simulink model "cpm_jap_r2019a"  (R2019a)
settings: Solver=ode4  StartTime=0.0  StopTime=inf  FixedStep=StepSize  RelTol=1e-3  EnableMultiTasking=on
PostLoadFcn:
  | %% PARAMETER INITIALIZATION
  | modelname = gcs;
  | p = Simulink.Mask.get([modelname, '/CP Model']);
  | 
  | %% HEART
  | % Basal heart period, T0 (s):
  | p.Parameters(1,1).Value = '0.58';
  | %% Right atrium
  | % RA Compliance, Cra (ml/mmHg):
  | p.Parameters(1,2).Value = '31.25';
  | % RA Resistance, Rra (mmHg s/ml):
  | p.Parameters(1,3).Value = '0.0025';
  | % RA Unstressed volume, Vu_ra (ml):
  | p.Parameters(1,4).Value = '22';
  | %% Left atrium
  | % LA Compliance, Cla (ml/mmHg):
  | p.Parameters(1,5).Value = '19.23';
  | % LA Resistance, Rla (mmHg s/ml):
  | p.Parameters(1,6).Value = '0.0025';
  | % LA Unstressed volume, Vu_la (ml):
  | p.Parameters(1,7).Value = '22';
  | %% Right ventricle
  | % RV Resistance coefficient, kR_rv (s/ml):
  | p.Parameters(1,8).Value = '0.0014';
  | % RV free wall End-systolic maximal elastance, Emax_rvf0 (mmHg/ml):
  | p.Parameters(1,9).Value = '1.412';
  | % RV free wall End-systolic unstressed volume, Vu_rvf (ml):
  | p.Parameters(1,10).Value = '35.904';
  | % RV free wall End-diastolic pressure intercept, P0_rvf (mmHg):
  | p.Parameters(1,11).Value = '1.5';
  | % RV free wall End-diastolic elastance coefficient, kE_rvf (1/ml):
  | p.Parameters(1,12).Value = '0.011';
  | % RV free wall Contraction delay (s):
  | p.Parameters(1,13).Value = '0';
  | %% Left ventricle
  | % LV Resistance coefficient, kR_lv (s/ml):
  | p.Parameters(1,14).Value = '0.00037';
  | % LV free wall End-systolic maximal elastance, Emax_lvf0 (mmHg/ml):
  | p.Parameters(1,15).Value = '2.392';
  | % LV free wall End-systolic unstressed volume, Vu_lvf (ml):
  | p.Parameters(1,16).Value = '14.7576';
  | % LV free wall End-diastolic pressure intercept, P0_lvf (mmHg):
  | p.Parameters(1,17).Value = '1.5';
  | % LV free wall End-diastolic elastance coefficient, kE_lvf (1/ml):
  | p.Parameters(1,18).Value = '0.014';
  | % LV Contraction delay (s):
  | p.Parameters(1,19).Value = '0';
  | %% Septum
  | % Septal End-systolic maximal elastance, Emax_spt0 (mmHg/ml):
  | p.Parameters(1,20).Value = '32.4';
  | % Septal End-systolic unstressed volume, Vu_spt (ml):
  | p.Parameters(1,21).Value = '0';
  | % Septal End-diastolic pressure intercept, P0_spt (mmHg):
  | p.Parameters(1,22).Value = '1.11';
  | % Septal End-diastolic elastance coefficient, kE_spt (1/ml):
  | p.Parameters(1,23).Value = '0.175';
  | %% Pericardium
  | % Pericardial Unstressed volume, Vu_pcd (ml):
  | p.Parameters(1,24).Value = '200';
  | % Pericardial Pressure intercept, P0_pcd (mmHg):
  | ... (+188 lines)
InitFcn:
  | logFreq = 100; % logging frequency
  | StepSize = 5e-4; % simulation step size
  | 
  | %% PARAMETER INITIALIZATION
  | modelname = gcs;
  | p = Simulink.Mask.get([modelname, '/CP Model']);
  | 
  | %% HEART
  | % Basal heart period, T0 (s):
  | p.Parameters(1,1).Value = '0.58';
  | %% Right atrium
  | % RA Compliance, Cra (ml/mmHg):
  | p.Parameters(1,2).Value = '31.25';
  | % RA Resistance, Rra (mmHg s/ml):
  | p.Parameters(1,3).Value = '0.0025';
  | % RA Unstressed volume, Vu_ra (ml):
  | p.Parameters(1,4).Value = '22';
  | %% Left atrium
  | % LA Compliance, Cla (ml/mmHg):
  | p.Parameters(1,5).Value = '19.23';
  | % LA Resistance, Rla (mmHg s/ml):
  | p.Parameters(1,6).Value = '0.0025';
  | % LA Unstressed volume, Vu_la (ml):
  | p.Parameters(1,7).Value = '22';
  | %% Right ventricle
  | % RV Resistance coefficient, kR_rv (s/ml):
  | p.Parameters(1,8).Value = '0.0014';
  | % RV free wall End-systolic maximal elastance, Emax_rvf0 (mmHg/ml):
  | p.Parameters(1,9).Value = '1.412';
  | % RV free wall End-systolic unstressed volume, Vu_rvf (ml):
  | p.Parameters(1,10).Value = '35.904';
  | % RV free wall End-diastolic pressure intercept, P0_rvf (mmHg):
  | p.Parameters(1,11).Value = '1.5';
  | % RV free wall End-diastolic elastance coefficient, kE_rvf (1/ml):
  | p.Parameters(1,12).Value = '0.011';
  | % RV free wall Contraction delay (s):
  | p.Parameters(1,13).Value = '0';
  | %% Left ventricle
  | % LV Resistance coefficient, kR_lv (s/ml):
  | p.Parameters(1,14).Value = '0.00037';
  | % LV free wall End-systolic maximal elastance, Emax_lvf0 (mmHg/ml):
  | p.Parameters(1,15).Value = '2.392';
  | % LV free wall End-systolic unstressed volume, Vu_lvf (ml):
  | p.Parameters(1,16).Value = '14.7576';
  | % LV free wall End-diastolic pressure intercept, P0_lvf (mmHg):
  | p.Parameters(1,17).Value = '1.5';
  | % LV free wall End-diastolic elastance coefficient, kE_lvf (1/ml):
  | p.Parameters(1,18).Value = '0.014';
  | % LV Contraction delay (s):
  | p.Parameters(1,19).Value = '0';
  | %% Septum
  | % Septal End-systolic maximal elastance, Emax_spt0 (mmHg/ml):
  | p.Parameters(1,20).Value = '32.4';
  | % Septal End-systolic unstressed volume, Vu_spt (ml):
  | p.Parameters(1,21).Value = '0';
  | % Septal End-diastolic pressure intercept, P0_spt (mmHg):
  | p.Parameters(1,22).Value = '1.11';
  | % Septal End-diastolic elastance coefficient, kE_spt (1/ml):
  | p.Parameters(1,23).Value = '0.175';
  | %% Pericardium
  | ... (+191 lines)
StopFcn:
  | cpmResults = cpm_jap{1}.Values;
(part 2 of 2)

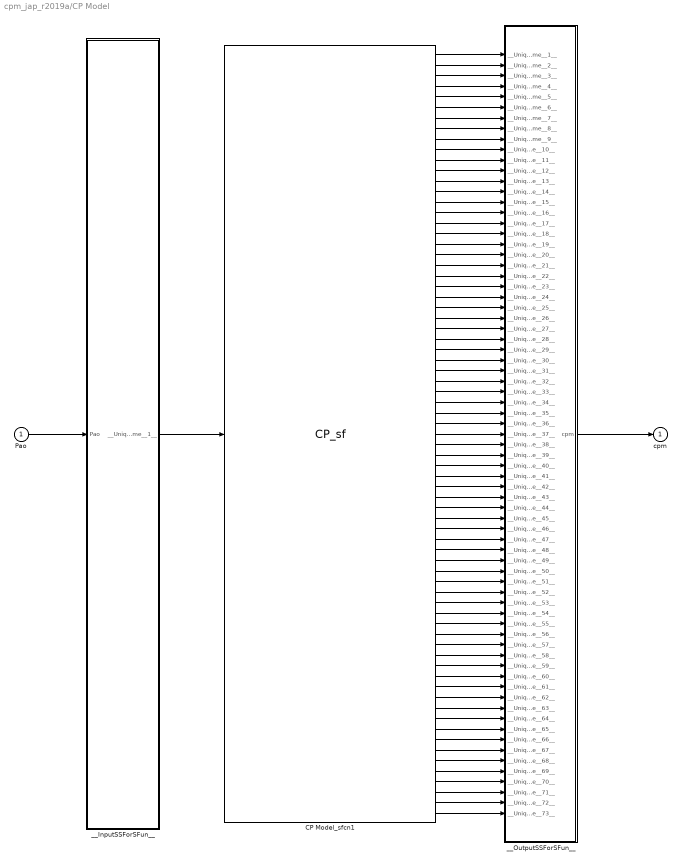
== system cpm_jap_r2019a/CP Model ==
  Pao : Inport  Unit=cmH2O
  CP Model_sfcn1 : S-Function  FunctionName=CP_sf  Parameters=sfcnParam1, sfcnParam2, sfcnParam3, sfcnParam4, sfcnParam5, sfcnParam6, sfcnParam7, sfcnParam8, sfcnParam9, sfcnParam10, sfcnParam11, sfcnParam12, sfcnParam13, sfcnParam14, sfcnParam15, sfcnParam16, sfcnParam17, sfcnParam18, sfcnParam19, sfcnParam20, sfcnParam21, sfcnParam22, sfcnParam23, sfcnParam24, sfcnParam25, sfcnParam26, sfcnParam27, sfcnParam28, sfcnParam29, sfcnParam30, sfcnParam31, sfcnParam32, sfcnParam33, sfcnParam34, sfcnParam35, sfcnParam36, sfcnParam37, sfcnParam38, sfcnParam39, sfcnParam40, sfcnParam41, sfcnParam42, sfcnParam43, sfcnParam44, sfcnParam45, sfcnParam46, sfcnParam47, sfcnParam48, sfcnParam49, sfcnParam50, sfcnParam51, sfcnParam52, sfcnParam53, sfcnParam54, sfcnParam55, sfcnParam56, sfcnParam57, sfcnParam58, sfcnParam59, sfcnParam60, sfcnParam61, sfcnParam62, sfcnParam63, sfcnParam64, sfcnParam65, sfcnParam66, sfcnParam67, sfcnParam68, sfcnParam69, sfcnParam70, sfcnParam71, sfcnParam72, sfcnParam73, sfcnParam74, sfcnParam75, sfcnParam76, sfcnParam77, sfcnParam78, sfcnParam79, sfcnParam80, sfcnParam81, sfcnParam82, sfcnParam83, sfcnParam84, sfcnParam85, sfcnParam86, sfcnParam87, sfcnParam88, sfcnParam89, sfcnParam90, sfcnParam91, sfcnParam92, sfcnParam93, sfcnParam94, sfcnParam95, sfcnParam96, sfcnParam97, sfcnParam98, sfcnParam99, sfcnParam100, sfcnParam101, sfcnParam102, sfcnParam103, sfcnParam104, sfcnParam105, sfcnParam106, sfcnParam107, sfcnParam108, sfcnParam109, sfcnParam110, sfcnParam111  SFunctionModules=""  SFunctionDeploymentMode=off  EnableBusSupport=off  SFcnStateName=DWORK0  mask{rtw_sf_name=CP_sf, showVar=off, sfcnParam1=sfcnParam1, sfcnParam2=sfcnParam2, sfcnParam3=sfcnParam3, sfcnParam4=sfcnParam4, sfcnParam5=sfcnParam5, sfcnParam6=sfcnParam6, sfcnParam7=sfcnParam7, sfcnParam8=sfcnParam8, sfcnParam9=sfcnParam9, sfcnParam10=sfcnParam10, sfcnParam11=sfcnParam11, sfcnParam12=sfcnParam12, sfcnParam13=sfcnParam13, sfcnParam14=sfcnParam14, sfcnParam15=sfcnParam15, sfcnParam16=sfcnParam16, sfcnParam17=sfcnParam17, sfcnParam18=sfcnParam18, sfcnParam19=sfcnParam19, sfcnParam20=sfcnParam20, sfcnParam21=sfcnParam21, sfcnParam22=sfcnParam22, sfcnParam23=sfcnParam23, sfcnParam24=2.25, sfcnParam25=sfcnParam25, sfcnParam26=sfcnParam26, sfcnParam27=sfcnParam27, sfcnParam28=sfcnParam28, sfcnParam29=sfcnParam29, sfcnParam30=sfcnParam30, sfcnParam31=sfcnParam31, sfcnParam32=sfcnParam32, sfcnParam33=sfcnParam33, sfcnParam34=sfcnParam34, sfcnParam35=sfcnParam35, sfcnParam36=sfcnParam36, sfcnParam37=sfcnParam37, sfcnParam38=sfcnParam38, sfcnParam39=sfcnParam39, sfcnParam40=sfcnParam40, sfcnParam41=sfcnParam41, sfcnParam42=sfcnParam42, sfcnParam43=sfcnParam43, sfcnParam44=sfcnParam44, sfcnParam45=sfcnParam45, sfcnParam46=sfcnParam46, sfcnParam47=sfcnParam47, sfcnParam48=sfcnParam48, sfcnParam49=sfcnParam49, sfcnParam50=sfcnParam50, sfcnParam51=sfcnParam51, sfcnParam52=sfcnParam52, sfcnParam53=sfcnParam53, sfcnParam54=sfcnParam54, sfcnParam55=sfcnParam55, sfcnParam56=sfcnParam56, sfcnParam57=sfcnParam57, sfcnParam58=sfcnParam58, sfcnParam59=sfcnParam59, sfcnParam60=sfcnParam60, sfcnParam61=sfcnParam61, sfcnParam62=sfcnParam62, sfcnParam63=sfcnParam63, sfcnParam64=sfcnParam64, sfcnParam65=sfcnParam65, sfcnParam66=sfcnParam66, sfcnParam67=sfcnParam67, sfcnParam68=sfcnParam68, sfcnParam69=sfcnParam69, sfcnParam70=sfcnParam70, sfcnParam71=sfcnParam71, sfcnParam72=0, sfcnParam73=sfcnParam73, sfcnParam74=sfcnParam74, sfcnParam75=sfcnParam75, sfcnParam76=sfcnParam76, sfcnParam77=sfcnParam77, sfcnParam78=sfcnParam78, sfcnParam79=sfcnParam79, sfcnParam80=sfcnParam80, sfcnParam81=sfcnParam81, sfcnParam82=sfcnParam82, sfcnParam83=sfcnParam83, sfcnParam84=sfcnParam84, sfcnParam85=sfcnParam85, sfcnParam86=sfcnParam86, sfcnParam87=sfcnParam87, sfcnParam88=sfcnParam88, sfcnParam89=sfcnParam89, sfcnParam90=sfcnParam90, sfcnParam91=sfcnParam91, sfcnParam92=sfcnParam92, sfcnParam93=sfcnParam93, sfcnParam94=sfcnParam94, sfcnParam95=sfcnParam95, sfcnParam96=0, sfcnParam97=sfcnParam97, sfcnParam98=sfcnParam98, sfcnParam99=sfcnParam99, sfcnParam100=sfcnParam100, sfcnParam101=sfcnParam101, sfcnParam102=sfcnParam102, sfcnParam103=sfcnParam103, sfcnParam104=sfcnParam104, sfcnParam105=sfcnParam105, sfcnParam106=sfcnParam106, sfcnParam107=sfcnParam107, sfcnParam108=sfcnParam108, sfcnParam109=sfcnParam109, sfcnParam110=sfcnParam110, sfcnParam111=sfcnParam111}
      mask prompts: rtw_sf_name "Simulink:masks:GenSFuncName_MP"; showVar "Simulink:masks:GenSFuncShowModuleList_MP"; sfcnParam1 "BreathAmp:"; sfcnParam2 "BreathFreq:"; sfcnParam3 "CL:"; sfcnParam4 "C_cw:"; sfcnParam5 "C_vc:"; sfcnParam6 "Cep:"; sfcnParam7 "Cev:"; sfcnParam8 "Cla:"; sfcnParam9 "ConsCO2Exspl:"; sfcnParam10 "ConsCO2Spl:"; sfcnParam11 "ConsO2Exspl:"; sfcnParam12 "ConsO2Spl:"; sfcnParam13 "Cpa:"; sfcnParam14 "Cpp_tot:"; sfcnParam15 "Cpv:"; sfcnParam16 "Cra:"; sfcnParam17 "Csa:"; sfcnParam18 "Csp:"; sfcnParam19 "Csv:"; sfcnParam20 "Ees_spt0:"; sfcnParam21 "Emax_lvf0:"; sfcnParam22 "Emax_rvf0:"; sfcnParam23 "ExsplVolume:"; sfcnParam24 "FRCnom:"; sfcnParam25 "FiCO2:"; sfcnParam26 "FiO2:"; sfcnParam27 "Gc_A_up:"; sfcnParam28 "Gc_f_up:"; sfcnParam29 "Gp_A_up:"; sfcnParam30 "Gp_f_up:"; sfcnParam31 "Gsr:"; sfcnParam32 "IEratio:"; sfcnParam33 "Lpa:"; sfcnParam34 "Lsa:"; sfcnParam35 "P0_lvf:"; sfcnParam36 "P0_pcd:"; sfcnParam37 "P0_rvf:"; sfcnParam38 "P0_spt:"; sfcnParam39 "PO2sh:"; sfcnParam40 "PO2sp:"; sfcnParam41 "PO2sv:"; sfcnParam42 "PaCO2n:"; sfcnParam43 "Pn:"; sfcnParam44 "RL:"; sfcnParam45 "R_vc_0:"; sfcnParam46 "Rep_0:"; sfcnParam47 "Ret:"; sfcnParam48 "Rev:"; sfcnParam49 "Rla:"; sfcnParam50 "Rpa:"; sfcnParam51 "Rpp_tot:"; sfcnParam52 "Rpv:"; sfcnParam53 "Rra:"; sfcnParam54 "Rsa:"; sfcnParam55 "Rsp_0:"; sfcnParam56 "Rsv:"; sfcnParam57 "SplVolume:"; sfcnParam58 "T0:"; sfcnParam59 "V0_pcd:"; sfcnParam60 "V0_spt:"; sfcnParam61 "V_pcd:"; sfcnParam62 "Vdead:"; sfcnParam63 "Vt:"; sfcnParam64 "Vu_L:"; sfcnParam65 "Vu_cw:"; sfcnParam66 "Vu_ep:"; sfcnParam67 "Vu_ev0:"; sfcnParam68 "Vu_la:"; sfcnParam69 "Vu_lvf:"; sfcnParam70 "Vu_pa:"; sfcnParam71 "Vu_pp:"; sfcnParam72 "Vu_ps:"; sfcnParam73 "Vu_pv:"; sfcnParam74 "Vu_ra:"; sfcnParam75 "Vu_rvf:"; sfcnParam76 "Vu_sa:"; sfcnParam77 "Vu_sp:"; sfcnParam78 "Vu_sv0:"; sfcnParam79 "Vu_vc:"; sfcnParam80 "Wbsh:"; sfcnParam81 "Wbsp:"; sfcnParam82 "Wbsv:"; sfcnParam83 "Wpcsh:"; sfcnParam84 "Wpcsp:"; sfcnParam85 "Wpcsv:"; sfcnParam86 "Wpcv:"; sfcnParam87 "Wsrsh:"; sfcnParam88 "Wsrsp:"; sfcnParam89 "Wsrsv:"; sfcnParam90 "Wsrv:"; sfcnParam91 "fapcn:"; sfcnParam92 "gccsh:"; sfcnParam93 "gccsp:"; sfcnParam94 "gccsv:"; sfcnParam95 "infusionDur:"; sfcnParam96 "kBloodLoss:"; sfcnParam97 "kE_lvf:"; sfcnParam98 "kE_rvf:"; sfcnParam99 "kRL_out:"; sfcnParam100 "kR_lv:"; sfcnParam101 "kR_rv:"; sfcnParam102 "kab:"; sfcnParam103 "kev:"; sfcnParam104 "lambda_pcd:"; sfcnParam105 "lambda_spt:"; sfcnParam106 "lvContractionDelay:"; sfcnParam107 "passivePatient:"; sfcnParam108 "pumpFlag:"; sfcnParam109 "rvContractionDelay:"; sfcnParam110 "sh:"; sfcnParam111 "volumeInfused:"
      mask help: Simulink:masks:GenSFuncDesc_MD
      mask init:
      | displist = '';
      | if ~strcmp(get_param(gcb, 'FunctionName'), rtw_sf_name);
      |   set_param(gcb, 'FunctionName', rtw_sf_name);
      | end
      | % Check if we are generating code
      | rtw_mode = false;
      | if strcmpi(get_param(bdroot(gcb),'SimulationStatus'),'Initializing')
      | 	rtw_mode = strcmpi(get_param(bdroot(gcb),'BuildingRTWCode'),'on') && ...
      | 		~strcmpi(get_param(bdroot(gcb),'TargetStyle'),'SimulationTarget');
      | end
      | if showVar || rtw_mode
      | 	if exist('rtwsfunc') == 2 | exist('rtwsfunc') == 6
      | 		tmplist = rtwsfunc(rtw_sf_name,gcb);
      | 		tmplist = DAStudio.message('Simulink:masks:GenSFuncListOfModules_IC', tmplist);
      | 	elseif showVar
      | 		tmplist1 = DAStudio.message('Simulink:masks:GenSFuncListOfModules_IC', '');
      |         tmplist2 = DAStudio.message('Simulink:masks:GenSFuncNotLicensed_IC');
      |         tmplist = [tmplist1 tmplist2];
      |  	end
      | end
      | if showVar
      |   displist = tmplist;
      | end
      settings: SFcnIsStateOwnerBlock=on
      settings: CopyFcn=|
      | if ~strcmp(get_param(gcb,'Linkstatus'),'none') && ...
      | ~strcmp(get_param(gcb,'Linkstatus'),'implicit')
      |   set_param(gcb,'LinkStatus','none');
      | end
      mask Help: eval('feval(''rtwprivate'',''rtwhelpview'',''rtw_sfcn_block'')');
      mask Display:
      | port_label('input',1,'Pao');
      | port_label('output',1,'Air flow');
      | port_label('output',2,'Pmus');
      | port_label('output',3,'Pao');
      | port_label('output',4,'PA');
      | port_label('output',5,'Ppl');
      | port_label('output',6,'V_T');
      | port_label('output',7,'V_L');
      | port_label('output',8,'Ve');
      | port_label('output',9,'RR');
      | port_label('output',10,'WOB');
      | port_label('output',11,'POB');
      | port_label('output',12,'PaO2');
      | port_label('output',13,'PaCO2');
      | port_label('output',14,'PAO2');
      | port_label('output',15,'PACO2');
      | port_label('output',16,'SaO2');
      | port_label('output',17,'ETCO2');
      | port_label('output',18,'fab');
      | port_label('output',19,'fapc');
      | port_label('output',20,'fasr');
      | port_label('output',21,'fsh');
      | port_label('output',22,'fsp');
      | port_label('output',23,'fsv');
      | port_label('output',24,'fev');
      | port_label('output',25,'Psa');
      | port_label('output',26,'Psa_sys');
      | port_label('output',27,'Psa_dias');
      | port_label('output',28,'Psa_mean');
      | port_label('output',29,'PP');
      | port_label('output',30,'DPP');
      | port_label('output',31,'Ppa');
      | port_label('output',32,'Ppa_sys');
      | port_label('output',33,'Ppa_dias');
      | port_label('output',34,'Ppa_mean');
      | port_label('output',35,'Pla');
      | port_label('output',36,'Pra');
      | port_label('output',37,'Plv');
      | port_label('output',38,'Prv');
      | port_label('output',39,'CO');
      | port_label('output',40,'CO_mean');
      | port_label('output',41,'HR');
      | port_label('output',42,'HR_mean');
      | port_label('output',43,'SV');
      | port_label('output',44,'SV_mean');
      | port_label('output',45,'SVI');
      | port_label('output',46,'SVI_mean');
      | port_label('output',47,'CI');
      | port_label('output',48,'CI_mean');
      | port_label('output',49,'phi');
      | port_label('output',50,'Vlv');
      | port_label('output',51,'Vlvf');
      | port_label('output',52,'Vrv');
      | port_label('output',53,'Vrvf');
      | port_label('output',54,'LVEF');
      | port_label('output',55,'LVESV');
      | port_label('output',56,'LVEDV');
      | port_label('output',57,'RVEF');
      | port_label('output',58,'RVESV');
      | port_label('output',59,'RVEDV');
      | port_label('output',60,'Qlvo');
      | port_label('output',61,'Qrvo');
      | port_label('output',62,'Pperi');
      | port_label('output',63,'Vspt');
      | port_label('output',64,'Vblood_thorax');
      | port_label('output',65,'Vblood_t');
      | port_label('output',66,'Emax_rvf');
      | port_label('output',67,'Emax_lvf');
      | port_label('output',68,'Emax_spt');
      | port_label('output',69,'Rsp');
      | port_label('output',70,'Rep');
      | port_label('output',71,'Vu_sv');
      | port_label('output',72,'Vu_ev');
      | port_label('output',73,'T');
  __InputSSForSFun__ : Subsystem
  __OutputSSForSFun__ : Subsystem
  cpm : Outport
  wires:
  Pao/1 -> __InputSSForSFun__/1(Pao)
  __InputSSForSFun__/1(__UniqueOutportName__1__) -> CP Model_sfcn1/1
  CP Model_sfcn1/1 -> __OutputSSForSFun__/1(__UniqueInportName__1__)
  CP Model_sfcn1/2 -> __OutputSSForSFun__/2(__UniqueInportName__2__)
  CP Model_sfcn1/3 -> __OutputSSForSFun__/3(__UniqueInportName__3__)
  CP Model_sfcn1/4 -> __OutputSSForSFun__/4(__UniqueInportName__4__)
  CP Model_sfcn1/5 -> __OutputSSForSFun__/5(__UniqueInportName__5__)
  CP Model_sfcn1/6 -> __OutputSSForSFun__/6(__UniqueInportName__6__)
  CP Model_sfcn1/7 -> __OutputSSForSFun__/7(__UniqueInportName__7__)
  CP Model_sfcn1/8 -> __OutputSSForSFun__/8(__UniqueInportName__8__)
  CP Model_sfcn1/9 -> __OutputSSForSFun__/9(__UniqueInportName__9__)
  CP Model_sfcn1/10 -> __OutputSSForSFun__/10(__UniqueInportName__10__)
  CP Model_sfcn1/11 -> __OutputSSForSFun__/11(__UniqueInportName__11__)
  CP Model_sfcn1/12 -> __OutputSSForSFun__/12(__UniqueInportName__12__)
  CP Model_sfcn1/13 -> __OutputSSForSFun__/13(__UniqueInportName__13__)
  CP Model_sfcn1/14 -> __OutputSSForSFun__/14(__UniqueInportName__14__)
  CP Model_sfcn1/15 -> __OutputSSForSFun__/15(__UniqueInportName__15__)
  CP Model_sfcn1/16 -> __OutputSSForSFun__/16(__UniqueInportName__16__)
  CP Model_sfcn1/17 -> __OutputSSForSFun__/17(__UniqueInportName__17__)
  CP Model_sfcn1/18 -> __OutputSSForSFun__/18(__UniqueInportName__18__)
  CP Model_sfcn1/19 -> __OutputSSForSFun__/19(__UniqueInportName__19__)
  CP Model_sfcn1/20 -> __OutputSSForSFun__/20(__UniqueInportName__20__)
  CP Model_sfcn1/21 -> __OutputSSForSFun__/21(__UniqueInportName__21__)
  CP Model_sfcn1/22 -> __OutputSSForSFun__/22(__UniqueInportName__22__)
  CP Model_sfcn1/23 -> __OutputSSForSFun__/23(__UniqueInportName__23__)
  CP Model_sfcn1/24 -> __OutputSSForSFun__/24(__UniqueInportName__24__)
  CP Model_sfcn1/25 -> __OutputSSForSFun__/25(__UniqueInportName__25__)
  CP Model_sfcn1/26 -> __OutputSSForSFun__/26(__UniqueInportName__26__)
  CP Model_sfcn1/27 -> __OutputSSForSFun__/27(__UniqueInportName__27__)
  CP Model_sfcn1/28 -> __OutputSSForSFun__/28(__UniqueInportName__28__)
  CP Model_sfcn1/29 -> __OutputSSForSFun__/29(__UniqueInportName__29__)
  CP Model_sfcn1/30 -> __OutputSSForSFun__/30(__UniqueInportName__30__)
  CP Model_sfcn1/31 -> __OutputSSForSFun__/31(__UniqueInportName__31__)
  CP Model_sfcn1/32 -> __OutputSSForSFun__/32(__UniqueInportName__32__)
  CP Model_sfcn1/33 -> __OutputSSForSFun__/33(__UniqueInportName__33__)
  CP Model_sfcn1/34 -> __OutputSSForSFun__/34(__UniqueInportName__34__)
  CP Model_sfcn1/35 -> __OutputSSForSFun__/35(__UniqueInportName__35__)
  CP Model_sfcn1/36 -> __OutputSSForSFun__/36(__UniqueInportName__36__)
  CP Model_sfcn1/37 -> __OutputSSForSFun__/37(__UniqueInportName__37__)
  CP Model_sfcn1/38 -> __OutputSSForSFun__/38(__UniqueInportName__38__)
  CP Model_sfcn1/39 -> __OutputSSForSFun__/39(__UniqueInportName__39__)
  CP Model_sfcn1/40 -> __OutputSSForSFun__/40(__UniqueInportName__40__)
  CP Model_sfcn1/41 -> __OutputSSForSFun__/41(__UniqueInportName__41__)
  CP Model_sfcn1/42 -> __OutputSSForSFun__/42(__UniqueInportName__42__)
  CP Model_sfcn1/43 -> __OutputSSForSFun__/43(__UniqueInportName__43__)
  CP Model_sfcn1/44 -> __OutputSSForSFun__/44(__UniqueInportName__44__)
  CP Model_sfcn1/45 -> __OutputSSForSFun__/45(__UniqueInportName__45__)
  CP Model_sfcn1/46 -> __OutputSSForSFun__/46(__UniqueInportName__46__)
  CP Model_sfcn1/47 -> __OutputSSForSFun__/47(__UniqueInportName__47__)
  CP Model_sfcn1/48 -> __OutputSSForSFun__/48(__UniqueInportName__48__)
  CP Model_sfcn1/49 -> __OutputSSForSFun__/49(__UniqueInportName__49__)
  CP Model_sfcn1/50 -> __OutputSSForSFun__/50(__UniqueInportName__50__)
  CP Model_sfcn1/51 -> __OutputSSForSFun__/51(__UniqueInportName__51__)
  CP Model_sfcn1/52 -> __OutputSSForSFun__/52(__UniqueInportName__52__)
  CP Model_sfcn1/53 -> __OutputSSForSFun__/53(__UniqueInportName__53__)
  CP Model_sfcn1/54 -> __OutputSSForSFun__/54(__UniqueInportName__54__)
  CP Model_sfcn1/55 -> __OutputSSForSFun__/55(__UniqueInportName__55__)
  CP Model_sfcn1/56 -> __OutputSSForSFun__/56(__UniqueInportName__56__)
  CP Model_sfcn1/57 -> __OutputSSForSFun__/57(__UniqueInportName__57__)
  CP Model_sfcn1/58 -> __OutputSSForSFun__/58(__UniqueInportName__58__)
  CP Model_sfcn1/59 -> __OutputSSForSFun__/59(__UniqueInportName__59__)
  CP Model_sfcn1/60 -> __OutputSSForSFun__/60(__UniqueInportName__60__)
  CP Model_sfcn1/61 -> __OutputSSForSFun__/61(__UniqueInportName__61__)
  CP Model_sfcn1/62 -> __OutputSSForSFun__/62(__UniqueInportName__62__)
  CP Model_sfcn1/63 -> __OutputSSForSFun__/63(__UniqueInportName__63__)
  CP Model_sfcn1/64 -> __OutputSSForSFun__/64(__UniqueInportName__64__)
  CP Model_sfcn1/65 -> __OutputSSForSFun__/65(__UniqueInportName__65__)
  CP Model_sfcn1/66 -> __OutputSSForSFun__/66(__UniqueInportName__66__)
  CP Model_sfcn1/67 -> __OutputSSForSFun__/67(__UniqueInportName__67__)
  CP Model_sfcn1/68 -> __OutputSSForSFun__/68(__UniqueInportName__68__)
  CP Model_sfcn1/69 -> __OutputSSForSFun__/69(__UniqueInportName__69__)
  CP Model_sfcn1/70 -> __OutputSSForSFun__/70(__UniqueInportName__70__)
  CP Model_sfcn1/71 -> __OutputSSForSFun__/71(__UniqueInportName__71__)
  CP Model_sfcn1/72 -> __OutputSSForSFun__/72(__UniqueInportName__72__)
  CP Model_sfcn1/73 -> __OutputSSForSFun__/73(__UniqueInportName__73__)
  __OutputSSForSFun__/1(cpm) -> cpm/1

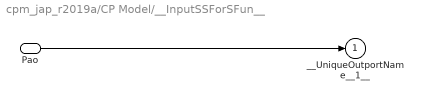
== system cpm_jap_r2019a/CP Model/__InputSSForSFun__ ==
  Pao : Inport  Unit=cmH2O
  __UniqueOutportName__1__ : Outport
  wires:
  Pao/1 -> __UniqueOutportName__1__/1

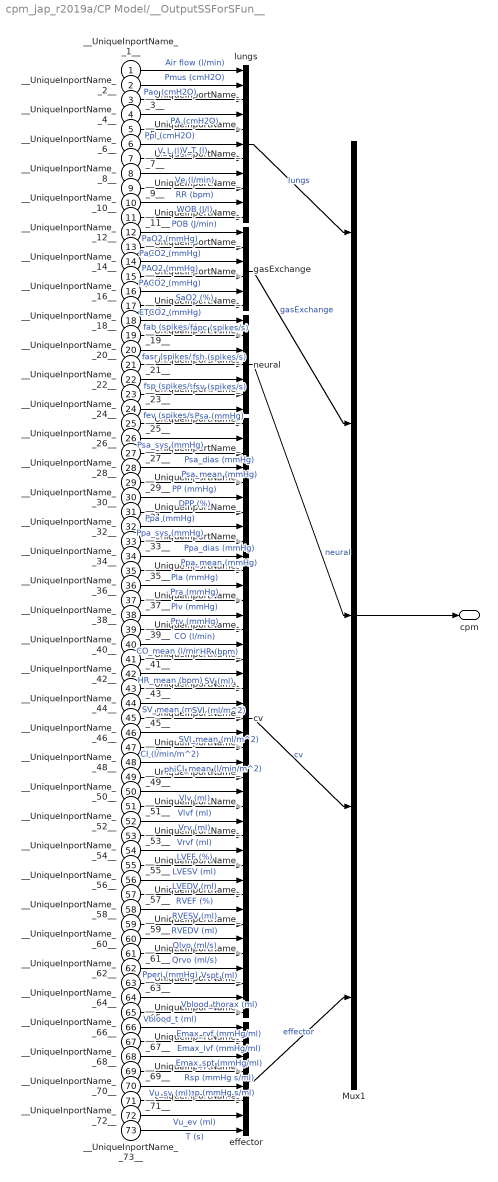
== system cpm_jap_r2019a/CP Model/__OutputSSForSFun__ ==
  __UniqueInportName__1__ : Inport  Unit=l/min
  __UniqueInportName__2__ : Inport  Port=2
  __UniqueInportName__3__ : Inport  Port=3
  __UniqueInportName__4__ : Inport  Port=4
  __UniqueInportName__5__ : Inport  Port=5
  __UniqueInportName__6__ : Inport  Port=6
  __UniqueInportName__7__ : Inport  Port=7
  __UniqueInportName__8__ : Inport  Port=8
  __UniqueInportName__9__ : Inport  Port=9
  __UniqueInportName__10__ : Inport  Port=10
  __UniqueInportName__11__ : Inport  Port=11
  __UniqueInportName__12__ : Inport  Port=12
  __UniqueInportName__13__ : Inport  Port=13
  __UniqueInportName__14__ : Inport  Port=14
  __UniqueInportName__15__ : Inport  Port=15
  __UniqueInportName__16__ : Inport  Port=16
  __UniqueInportName__17__ : Inport  Port=17
  __UniqueInportName__18__ : Inport  Port=18
  __UniqueInportName__19__ : Inport  Port=19
  __UniqueInportName__20__ : Inport  Port=20
  __UniqueInportName__21__ : Inport  Port=21
  __UniqueInportName__22__ : Inport  Port=22
  __UniqueInportName__23__ : Inport  Port=23
  __UniqueInportName__24__ : Inport  Port=24
  __UniqueInportName__25__ : Inport  Port=25
  __UniqueInportName__26__ : Inport  Port=26
  __UniqueInportName__27__ : Inport  Port=27
  __UniqueInportName__28__ : Inport  Port=28
  __UniqueInportName__29__ : Inport  Port=29
  __UniqueInportName__30__ : Inport  Port=30
  __UniqueInportName__31__ : Inport  Port=31
  __UniqueInportName__32__ : Inport  Port=32
  __UniqueInportName__33__ : Inport  Port=33
  __UniqueInportName__34__ : Inport  Port=34
  __UniqueInportName__35__ : Inport  Port=35
  __UniqueInportName__36__ : Inport  Port=36
  __UniqueInportName__37__ : Inport  Port=37
  __UniqueInportName__38__ : Inport  Port=38
  __UniqueInportName__39__ : Inport  Port=39
  __UniqueInportName__40__ : Inport  Port=40
  __UniqueInportName__41__ : Inport  Port=41
  __UniqueInportName__42__ : Inport  Port=42
  __UniqueInportName__43__ : Inport  Port=43
  __UniqueInportName__44__ : Inport  Port=44
  __UniqueInportName__45__ : Inport  Port=45
  __UniqueInportName__46__ : Inport  Port=46
  __UniqueInportName__47__ : Inport  Port=47
  __UniqueInportName__48__ : Inport  Port=48
  __UniqueInportName__49__ : Inport  Port=49
  __UniqueInportName__50__ : Inport  Port=50
  __UniqueInportName__51__ : Inport  Port=51
  __UniqueInportName__52__ : Inport  Port=52
  __UniqueInportName__53__ : Inport  Port=53
  __UniqueInportName__54__ : Inport  Port=54
  __UniqueInportName__55__ : Inport  Port=55
  __UniqueInportName__56__ : Inport  Port=56
  __UniqueInportName__57__ : Inport  Port=57
  __UniqueInportName__58__ : Inport  Port=58
  __UniqueInportName__59__ : Inport  Port=59
  __UniqueInportName__60__ : Inport  Port=60
  __UniqueInportName__61__ : Inport  Port=61
  __UniqueInportName__62__ : Inport  Port=62
  __UniqueInportName__63__ : Inport  Port=63
  __UniqueInportName__64__ : Inport  Port=64
  __UniqueInportName__65__ : Inport  Port=65
  __UniqueInportName__66__ : Inport  Port=66
  __UniqueInportName__67__ : Inport  Port=67
  __UniqueInportName__68__ : Inport  Port=68
  __UniqueInportName__69__ : Inport  Port=69
  __UniqueInportName__70__ : Inport  Port=70
  __UniqueInportName__71__ : Inport  Port=71
  __UniqueInportName__72__ : Inport  Port=72
  __UniqueInportName__73__ : Inport  Port=73
  Mux1 : BusCreator  Inputs=5
  cv : BusCreator  Inputs=41
  effector : BusCreator  Inputs=8
  gasExchange : BusCreator  Inputs=6
  lungs : BusCreator  Inputs=11
  neural : BusCreator  Inputs=7
  cpm : Outport
  wires:
  __UniqueInportName__1__/1 -> lungs/1  "Air flow (l/min)"
  __UniqueInportName__2__/1 -> lungs/2  "Pmus (cmH2O)"
  __UniqueInportName__3__/1 -> lungs/3  "Pao (cmH2O)"
  __UniqueInportName__4__/1 -> lungs/4  "PA (cmH2O)"
  __UniqueInportName__5__/1 -> lungs/5  "Ppl (cmH2O)"
  __UniqueInportName__6__/1 -> lungs/6  "V_T (l)"
  __UniqueInportName__7__/1 -> lungs/7  "V_L (l)"
  __UniqueInportName__8__/1 -> lungs/8  "Ve (l/min)"
  __UniqueInportName__9__/1 -> lungs/9  "RR (bpm)"
  __UniqueInportName__10__/1 -> lungs/10  "WOB (J/l)"
  __UniqueInportName__11__/1 -> lungs/11  "POB (J/min)"
  __UniqueInportName__12__/1 -> gasExchange/1  "PaO2 (mmHg)"
  __UniqueInportName__13__/1 -> gasExchange/2  "PaCO2 (mmHg)"
  __UniqueInportName__14__/1 -> gasExchange/3  "PAO2 (mmHg)"
  __UniqueInportName__15__/1 -> gasExchange/4  "PACO2 (mmHg)"
  __UniqueInportName__16__/1 -> gasExchange/5  "SaO2 (%)"
  __UniqueInportName__17__/1 -> gasExchange/6  "ETCO2 (mmHg)"
  __UniqueInportName__18__/1 -> neural/1  "fab (spikes/s)"
  __UniqueInportName__19__/1 -> neural/2  "fapc (spikes/s)"
  __UniqueInportName__20__/1 -> neural/3  "fasr (spikes/s)"
  __UniqueInportName__21__/1 -> neural/4  "fsh (spikes/s)"
  __UniqueInportName__22__/1 -> neural/5  "fsp (spikes/s)"
  __UniqueInportName__23__/1 -> neural/6  "fsv (spikes/s)"
  __UniqueInportName__24__/1 -> neural/7  "fev (spikes/s)"
  __UniqueInportName__25__/1 -> cv/1  "Psa (mmHg)"
  __UniqueInportName__26__/1 -> cv/2  "Psa_sys (mmHg)"
  __UniqueInportName__27__/1 -> cv/3  "Psa_dias (mmHg)"
  __UniqueInportName__28__/1 -> cv/4  "Psa_mean (mmHg)"
  __UniqueInportName__29__/1 -> cv/5  "PP (mmHg)"
  __UniqueInportName__30__/1 -> cv/6  "DPP (%)"
  __UniqueInportName__31__/1 -> cv/7  "Ppa (mmHg)"
  __UniqueInportName__32__/1 -> cv/8  "Ppa_sys (mmHg)"
  __UniqueInportName__33__/1 -> cv/9  "Ppa_dias (mmHg)"
  __UniqueInportName__34__/1 -> cv/10  "Ppa_mean (mmHg)"
  __UniqueInportName__35__/1 -> cv/11  "Pla (mmHg)"
  __UniqueInportName__36__/1 -> cv/12  "Pra (mmHg)"
  __UniqueInportName__37__/1 -> cv/13  "Plv (mmHg)"
  __UniqueInportName__38__/1 -> cv/14  "Prv (mmHg)"
  __UniqueInportName__39__/1 -> cv/15  "CO (l/min)"
  __UniqueInportName__40__/1 -> cv/16  "CO_mean (l/min)"
  __UniqueInportName__41__/1 -> cv/17  "HR (bpm)"
  __UniqueInportName__42__/1 -> cv/18  "HR_mean (bpm)"
  __UniqueInportName__43__/1 -> cv/19  "SV (ml)"
  __UniqueInportName__44__/1 -> cv/20  "SV_mean (ml)"
  __UniqueInportName__45__/1 -> cv/21  "SVI (ml/m^2)"
  __UniqueInportName__46__/1 -> cv/22  "SVI_mean (ml/m^2)"
  __UniqueInportName__47__/1 -> cv/23  "CI (l/min/m^2)"
  __UniqueInportName__48__/1 -> cv/24  "CI_mean (l/min/m^2)"
  __UniqueInportName__49__/1 -> cv/25  "phi"
  __UniqueInportName__50__/1 -> cv/26  "Vlv (ml)"
  __UniqueInportName__51__/1 -> cv/27  "Vlvf (ml)"
  __UniqueInportName__52__/1 -> cv/28  "Vrv (ml)"
  __UniqueInportName__53__/1 -> cv/29  "Vrvf (ml)"
  __UniqueInportName__54__/1 -> cv/30  "LVEF (%)"
  __UniqueInportName__55__/1 -> cv/31  "LVESV (ml)"
  __UniqueInportName__56__/1 -> cv/32  "LVEDV (ml)"
  __UniqueInportName__57__/1 -> cv/33  "RVEF (%)"
  __UniqueInportName__58__/1 -> cv/34  "RVESV (ml)"
  __UniqueInportName__59__/1 -> cv/35  "RVEDV (ml)"
  __UniqueInportName__60__/1 -> cv/36  "Qlvo (ml/s)"
  __UniqueInportName__61__/1 -> cv/37  "Qrvo (ml/s)"
  __UniqueInportName__62__/1 -> cv/38  "Pperi (mmHg)"
  __UniqueInportName__63__/1 -> cv/39  "Vspt (ml)"
  __UniqueInportName__64__/1 -> cv/40  "Vblood_thorax (ml)"
  __UniqueInportName__65__/1 -> cv/41  "Vblood_t (ml)"
  __UniqueInportName__66__/1 -> effector/1  "Emax_rvf (mmHg/ml)"
  __UniqueInportName__67__/1 -> effector/2  "Emax_lvf (mmHg/ml)"
  __UniqueInportName__68__/1 -> effector/3  "Emax_spt (mmHg/ml)"
  __UniqueInportName__69__/1 -> effector/4  "Rsp (mmHg s/ml)"
  __UniqueInportName__70__/1 -> effector/5  "Rep (mmHg s/ml)"
  __UniqueInportName__71__/1 -> effector/6  "Vu_sv (ml)"
  __UniqueInportName__72__/1 -> effector/7  "Vu_ev (ml)"
  __UniqueInportName__73__/1 -> effector/8  "T (s)"
  lungs/1 -> Mux1/1  "lungs"
  gasExchange/1 -> Mux1/2  "gasExchange"
  neural/1 -> Mux1/3  "neural"
  cv/1 -> Mux1/4  "cv"
  effector/1 -> Mux1/5  "effector"
  Mux1/1 -> cpm/1
